simulink model "TRNG_model"  (R2024a)
settings: Solver=VariableStepAuto  StartTime=0.0  StopTime=time  RelTol=1e-3
values from neighbouring files (symbols this model uses):
  ts = time/n    [Load_data.m]
libraries: simulink_extras x2
settings Model: Creator=Asep Nugroho  LastModifiedBy=Asep Nugroho
settings RTWCC: GPUComputeCapability=3.5

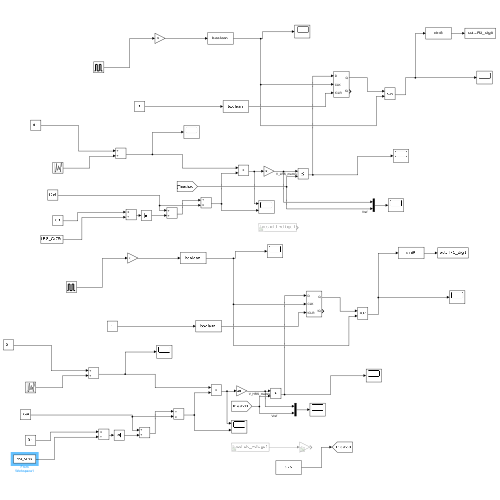
[thumbnail: Simulink's stored preview of the top-level diagram]
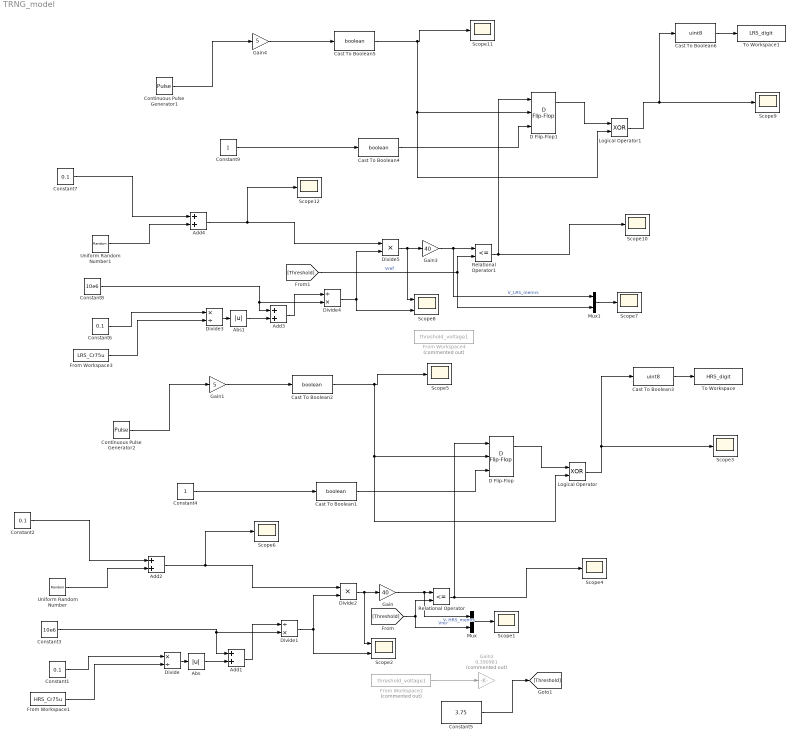
== system TRNG_model ==
  Abs : Abs  SaturateOnIntegerOverflow=off
  Abs1 : Abs  SaturateOnIntegerOverflow=off
  Add{1..4} (4 alike) : Sum
  Cast To Boolean{1..2,4..5} (4 alike) : DataTypeConversion  OutDataTypeStr=boolean  SaturateOnIntegerOverflow=off  RndMeth=Floor
  Cast To Boolean3 : DataTypeConversion  OutDataTypeStr=uint8  SaturateOnIntegerOverflow=off  RndMeth=Floor
  Cast To Boolean6 : DataTypeConversion  OutDataTypeStr=uint8  SaturateOnIntegerOverflow=off  RndMeth=Floor
  Constant1 : Constant  Value=0.1  SampleTime=-1
  Constant2 : Constant  Value=0.1
  Constant3 : Constant  Value=10e6  SampleTime=ts
  Constant4 : Constant
  Constant5 : Constant  Value=3.75
  Constant6 : Constant  Value=0.1  SampleTime=-1
  Constant7 : Constant  Value=0.1
  Constant8 : Constant  Value=10e6  SampleTime=ts
  Constant9 : Constant
  Continuous Pulse Generator1 : DiscretePulseGenerator  PulseType=Time based  Amplitude=0.1  Period=ts*0.3  PulseWidth=40
  Continuous Pulse Generator2 : DiscretePulseGenerator  PulseType=Time based  Amplitude=0.1  Period=ts*0.3  PulseWidth=40
  D Flip-Flop : simulink_extras/Flip Flops/D Flip-Flop
  D Flip-Flop1 : simulink_extras/Flip Flops/D Flip-Flop
  Divide : Product  Inputs=*/
  Divide1 : Product  Inputs=/*
  Divide2 : Product  Inputs=**
  Divide3 : Product  Inputs=*/
  Divide4 : Product  Inputs=/*
  Divide5 : Product  Inputs=**
  From Workspace1 : FromWorkspace  VariableName=HRS_Cr75u  SampleTime=ts  ZeroCross=off
  From Workspace2 : FromWorkspace  Commented=on  VariableName=threshold_voltage1  SampleTime=ts  ZeroCross=off
  From Workspace3 : FromWorkspace  VariableName=LRS_Cr75u  SampleTime=ts  ZeroCross=off
  From Workspace4 : FromWorkspace  Commented=on  VariableName=threshold_voltage1  SampleTime=ts  ZeroCross=off
  Gain : Gain  Gain=40
  Gain1 : Gain  Gain=5
  Gain2 : Gain  Commented=on  Gain=0.390981
  Gain3 : Gain  Gain=40
  Gain4 : Gain  Gain=5
  Logical Operator : Logic  Operator=XOR  AllPortsSameDT=off  OutDataTypeStr=boolean
  Logical Operator1 : Logic  Operator=XOR  AllPortsSameDT=off  OutDataTypeStr=boolean
  Mux : Mux  Inputs=2
  Mux1 : Mux  Inputs=2
  Relational Operator : RelationalOperator  Operator=<=  OutDataTypeStr=boolean  RndMeth=Simplest  InputSameDT=off
  Relational Operator1 : RelationalOperator  Operator=<=  OutDataTypeStr=boolean  RndMeth=Simplest  InputSameDT=off
  Scope{1,3..7,9..12} (10 alike) : Scope
  Scope2 : Scope  NumInputPorts=2
  Scope8 : Scope  NumInputPorts=2
  To Workspace : ToWorkspace  VariableName=HRS_digit  SampleTime=ts
      settings: Save2DSignal=2-D array (concatenate along first dimension)
  To Workspace1 : ToWorkspace  VariableName=LRS_digit  SampleTime=ts
      settings: Save2DSignal=2-D array (concatenate along first dimension)
  Uniform Random Number : UniformRandomNumber  Minimum=-0.001  Maximum=0.001  SampleTime=ts
  Uniform Random Number1 : UniformRandomNumber  Minimum=-0.001  Maximum=0.001  SampleTime=ts
  wires:
  Add1/1 -> Divide1/1
  Divide/1 -> Abs/1
  [Threshold] -> Relational Operator/2, Mux/2  "Vref"
  Constant3/1 -> Add1/1, Divide1/2
  Continuous Pulse Generator2/1 -> Gain1/1
  Constant2/1 -> Add2/1
  Divide1/1 -> Scope2/2, Divide2/2
  Logical Operator/1 -> Cast To Boolean3/1, Scope3/1
  Add2/1 -> Scope6/1, Divide2/1
  Gain/1 -> Mux/1, Relational Operator/1  "V_HRS_memrs"
  Constant4/1 -> Cast To Boolean1/1
  D Flip-Flop/1 -> Logical Operator/1
  Cast To Boolean1/1 -> D Flip-Flop/3
  Cast To Boolean2/1 -> Logical Operator/2, D Flip-Flop/2, Scope5/1
  Divide2/1 -> Scope2/1, Gain/1
  From Workspace2/1 -> Gain2/1
  Constant5/1 -> [Threshold]
  Gain1/1 -> Cast To Boolean2/1
  Cast To Boolean3/1 -> To Workspace/1
  Relational Operator/1 -> D Flip-Flop/1, Scope4/1
  Abs/1 -> Add1/2
  Uniform Random Number/1 -> Add2/2
  Constant1/1 -> Divide/1
  From Workspace1/1 -> Divide/2
  From Workspace3/1 -> Divide3/2
  Uniform Random Number1/1 -> Add4/2
  Cast To Boolean6/1 -> To Workspace1/1
  Gain4/1 -> Cast To Boolean5/1
  Relational Operator1/1 -> D Flip-Flop1/1, Scope10/1
  Cast To Boolean4/1 -> D Flip-Flop1/3
  Cast To Boolean5/1 -> Logical Operator1/2, D Flip-Flop1/2, Scope11/1
  Divide5/1 -> Scope8/1, Gain3/1
  D Flip-Flop1/1 -> Logical Operator1/1
  Add4/1 -> Scope12/1, Divide5/1
  Constant9/1 -> Cast To Boolean4/1
  Continuous Pulse Generator1/1 -> Gain4/1
  Divide4/1 -> Scope8/2, Divide5/2
  Gain3/1 -> Mux1/1, Relational Operator1/1  "V_LRS_memrs"
  Constant6/1 -> Divide3/1
  Logical Operator1/1 -> Cast To Boolean6/1, Scope9/1
  Constant7/1 -> Add4/1
  Divide3/1 -> Abs1/1
  Add3/1 -> Divide4/1
  Abs1/1 -> Add3/2
  Constant8/1 -> Divide4/2, Add3/1
  Mux/1 -> Scope1/1
  [Threshold] -> Relational Operator1/2, Mux1/2  "Vref"
  Mux1/1 -> Scope7/1
